simulink model "nncontroller_3_50"  (R2021a)
settings: Solver=VariableStepAuto  StartTime=0.0  StopTime=10.0  RelTol=1e-3
libraries: neural x155
(part 8 of 8)

== system nncontroller_3_50/Feed-Forward Neural Network/Layer 4/Delays 1 ==
  "p{4}" : Inport  PortDimensions=50
      mask Display: e = 0.06;c1 = [120 230 180]/255;c2 = ([120 230 180]+0)/(256+128);c3 = ([120 230 180]+128)/(256+128);patch([0 1 1 0],[0 0 1 1],c1);patch([0 1 1 1-e 1-e 0+e],[0 0 1 1-e 0+e 0+e],c2);patch([0 0 1 1-e 0+e 0+e],[0 1 1 1-e 1-e 0+e],c3);plot([0 1 1 0 0],[0 0 1 1 0]);
  mux : Mux  Inputs=1
      mask Display: e = 0.06;c1 = [120 150 230]/255;c2 = ([120 150 230]+0)/383;c3 = ([120 150 230]+128)/383;patch([0 1 1 0],[0 0 1 1],c1);patch([0 1 1 1-e 1-e 0+e],[0 0 1 1-e 0+e 0+e],c2);patch([0 0 1 1-e 0+e 0+e],[0 1 1 1-e 1-e 0+e],c3);plot([0 1 1 0 0],[0 0 1 1 0]);disp('Mux')
  "pd{4,3}" : Outport
      mask Display: e = 0.06;c1 = [120 230 180]/255;c2 = ([120 230 180]+0)/(256+128);c3 = ([120 230 180]+128)/(256+128);patch([0 1 1 0],[0 0 1 1],c1);patch([0 1 1 1-e 1-e 0+e],[0 0 1 1-e 0+e 0+e],c2);patch([0 0 1 1-e 0+e 0+e],[0 1 1 1-e 1-e 0+e],c3);plot([0 1 1 0 0],[0 0 1 1 0]);
  wires:
  "p{4}"/1 -> mux/1
  mux/1 -> "pd{4,3}"/1

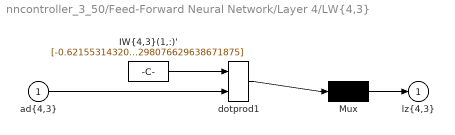
== system nncontroller_3_50/Feed-Forward Neural Network/Layer 4/LW{4,3} ==
  "ad{4,3}" : Inport  PortDimensions=50
      mask Display: e = 0.06;c1 = [120 230 180]/255;c2 = ([120 230 180]+0)/(256+128);c3 = ([120 230 180]+128)/(256+128);patch([0 1 1 0],[0 0 1 1],c1);patch([0 1 1 1-e 1-e 0+e],[0 0 1 1-e 0+e 0+e],c2);patch([0 0 1 1-e 0+e 0+e],[0 1 1 1-e 1-e 0+e],c3);plot([0 1 1 0 0],[0 0 1 1 0]);
  "IW{4,3}(1,:)'" : Constant  Value=[-0.621553143201879709778268079389818012714385986328125;0.7814466170737308647886720791575498878955841064453125;0.6381219856347921659533994898083619773387908935546875;-0.11187324505143703134990573744289577007293701171875;0.38863990484061716745856074339826591312885284423828125;0.01040766208472497685033619774230828625150024890899658203125;0.249282147379790430807844359151204116642475128173828125;-0.034124291878578905112817665212787687778472900390625;-0.11174429441240597837836645567222149111330509185791015625;-0.823607755593254164949712503585033118724822998046875;0.347703980543573043515692688743001781404018402099609375;-0.452460906868349166387588411453180015087127685546875;0.88196392410095747482756678436999209225177764892578125;0.88854540601630727092441475178929977118968963623046875;-0.32720475413273641951406034422689117491245269775390625;0.447145717685731136636917426585569046437740325927734375;-0.146439693243625157492715516127645969390869140625;-0.57805881442449968954377936825039796531200408935546875;0.4151732694670327017405497826985083520412445068359375;-0.274863680650872133082174286755616776645183563232421875;-0.474077193898417903472619627791573293507099151611328125;0.238796568586722823823720318614505231380462646484375;0.7912573483115672434706766580347903072834014892578125;-0.81714210026305822420766844516037963330745697021484375;-0.01502727199078297826151384697368484921753406524658203125;0.0788229415547052614243739299126900732517242431640625;-0.70318827770340475158405979527742601931095123291015625;-0.5505532682412093148371923234662972390651702880859375;-0.70871050996265816390717873218818567693233489990234375;0.963983672198847951761990771046839654445648193359375;0.2050938484799101624300732282790704630315303802490234375;0.92201864710671721514501086858217604458332061767578125;0.08431290322020561223137491424495237879455089569091796875;-0.339837348409870843024549458277761004865169525146484375;0.09916056196444920922683508024420007131993770599365234375;-0.894006206268517455981736929970793426036834716796875;-0.5766312426140196567558859896962530910968780517578125;-0.446148286439286945181947885430417954921722412109375;0.61648214253754163305387692162184976041316986083984375;-0.63635475826681020539155042570200748741626739501953125;-0.65242979620330476819844989222474396228790283203125;0.1905280579032486709678551051183603703975677490234375;0.231333159549040434654898490407504141330718994140625;-0.8734235402538141901374046938144601881504058837890625;0.46411616757972751212690809552441351115703582763671875;0.3492879573971132689536034376942552626132965087890625;0.050538396647102690195652030524797737598419189453125;0.13974627196960032193828737945295870304107666015625;-0.5067033558345672705769402455189265310764312744140625;0.93066457973218319477126669880817644298076629638671875]
      mask Display: e = 0.06;c1 = [120 150 230]/255;c2 = ([120 150 230]+0)/383;c3 = ([120 150 230]+128)/383;patch([0 1 1 0],[0 0 1 1],c1);patch([0 1 1 1-e 1-e 0+e],[0 0 1 1-e 0+e 0+e],c2);patch([0 0 1 1-e 0+e 0+e],[0 1 1 1-e 1-e 0+e],c3);plot([0 1 1 0 0],[0 0 1 1 0]);disp('weights');
  Mux : Mux  Inputs=1
      mask Display: e = 0.06;c1 = [120 150 230]/255;c2 = ([120 150 230]+0)/383;c3 = ([120 150 230]+128)/383;patch([0 1 1 0],[0 0 1 1],c1);patch([0 1 1 1-e 1-e 0+e],[0 0 1 1-e 0+e 0+e],c2);patch([0 0 1 1-e 0+e 0+e],[0 1 1 1-e 1-e 0+e],c3);plot([0 1 1 0 0],[0 0 1 1 0]);disp('Mux');
  dotprod1 : neural/Weight Functions/dotprod
  "lz{4,3}" : Outport
      mask Display: e = 0.06;c1 = [120 230 180]/255;c2 = ([120 230 180]+0)/(256+128);c3 = ([120 230 180]+128)/(256+128);patch([0 1 1 0],[0 0 1 1],c1);patch([0 1 1 1-e 1-e 0+e],[0 0 1 1-e 0+e 0+e],c2);patch([0 0 1 1-e 0+e 0+e],[0 1 1 1-e 1-e 0+e],c3);plot([0 1 1 0 0],[0 0 1 1 0]);
  wires:
  "IW{4,3}(1,:)'"/1 -> dotprod1/1
  "ad{4,3}"/1 -> dotprod1/2
  dotprod1/1 -> Mux/1
  Mux/1 -> "lz{4,3}"/1
